simulink model "sol4"  (R2018a)
settings: Solver=VariableStepAuto  StartTime=0.0  StopTime=30.0  RelTol=1e-3
settings Model: Creator=soutrik  LastModifiedBy=soutrik

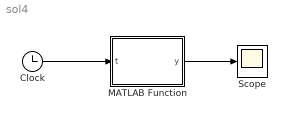
== system sol4 ==
  Clock : Clock
  MATLAB Function : MATLAB Function  TreatAsAtomicUnit=on
  Scope : Scope
  wires:
  Clock/1 -> MATLAB Function/1(t)
  MATLAB Function/1(y) -> Scope/1

== matlab function sol4/MATLAB Function ==
  data: t input; y output
function y = fcn(t)
y = exp(sin(t)) * exp(-0.15 * t);
end
